simulink model "sweep_testbench"  (Simulink 10.3)
settings: Solver=FixedStepDiscrete  StartTime=0.0  StopTime=swpctrl.trantime  FixedStep=1/Fs  RelTol=1e-3  EnableMultiTasking=on
undefined symbols (not defined in the file): Fs, input_dc, sinamp, sinfreq, swpctrl
libraries: dspsrcs4 x1
settings Model: Creator=amyles  LastModifiedBy=samir
settings DebuggingCC: SolverPrmCheckMsg=warning
settings ModelReferenceCC: ModelReferenceNumInstancesAllowed=Single

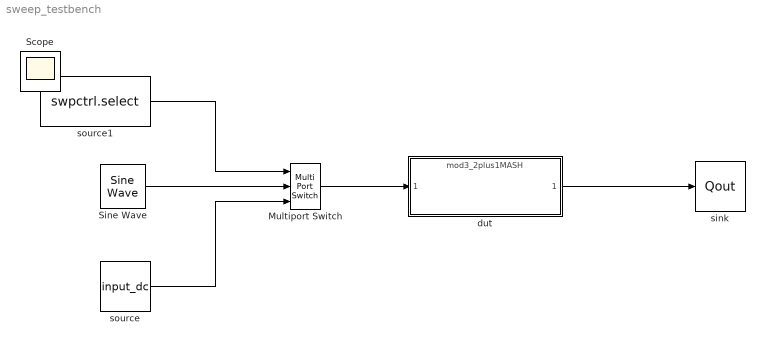
== system sweep_testbench ==
  Multiport Switch : MultiPortSwitch  Inputs=2
  Sine Wave : dspsrcs4/Sine Wave  Amplitude=sinamp  Frequency=sinfreq  Phase=0  SampleMode=Discrete  OutComplex=Real  CompMethod=Trigonometric fcn  TableSize=Speed  SampleTime=1/Fs  SamplesPerFrame=1  ResetState=Restart at time zero  OutputFrames=on  dataType=double  wordLen=16  udDataType=sfix(16)  fracBitsMode=Best precision  numFracBits=15  OutDataTypeStr=double  LastOutDataTypeStr=double
  dut : ModelReference  ModelNameDialog=mod3_2plus1MASH.mdl  SimulationMode=Normal  ModelReferenceVersion=17.4
  sink : ToWorkspace  VariableName=Qout  SampleTime=-1
      settings: MaxDataPoints=50000000
  source : Constant  Value=input_dc  SampleTime=1/Fs
  source1 : Constant  Value=swpctrl.select  SampleTime=1/Fs
  Scope : Scope
  wires:
  Sine Wave/1 -> Multiport Switch/2
  source/1 -> Multiport Switch/3
  source1/1 -> Multiport Switch/1
  dut/1 -> sink/1
  Multiport Switch/1 -> dut/1
